simulink model "LongLatDriveline"  (R2024b)
settings: Solver=FixedStepAuto  StartTime=0  StopTime=120  FixedStep=0.002  RelTol=1e-3
InitFcn:
  | load('waypoints.mat');
  | VehicleObj = Simulink.data.dictionary.open('./ModelData/VehicleData.sldd');
  | %dDataSectObj = getSection(myDictionaryObj,'Design Data');
StopFcn:
  | Plot_LateralModelErrorControl;
  | 
  | mdlWks = get_param(gcs, 'ModelWorkspace');
  | par_ToDrvDesigner = evalin(mdlWks, 'ToDrvDesigner');
  | 
  | if par_ToDrvDesigner.Value
  |     ExportdrivingScenario;
  | end
model workspace (MAT data in the model file):
  ToDrvDesigner = Simulink.Parameter
  ToDrvDesigner.Value = 1
  ToDrvDesigner.Complexity = 'real'
  ToDrvDesigner.Dimensions = [1 1]
  ToDrvDesigner.DataType = 'boolean'
values from neighbouring files (symbols this model uses):
  A_F = 2.341157    [VehicleData.sldd]
  C_af = 80000.0    [VehicleData.sldd]
  C_ar = 80000.0    [VehicleData.sldd]
  C_d = 0.24    [VehicleData.sldd]
  f = 0.01    [VehicleData.sldd]
  g = 9.81    [VehicleData.sldd]
  h_aero = 0.65    [VehicleData.sldd]
  h_gc = 0.65    [VehicleData.sldd]
  Iz = 2873.0    [VehicleData.sldd]
  lf = 1.1    [VehicleData.sldd]
  lr = 1.58    [VehicleData.sldd]
  m = 2238.932    [VehicleData.sldd]
  Nf = 2.0    [VehicleData.sldd]
  Nr = 2.0    [VehicleData.sldd]
  r_stat = 0.342    [VehicleData.sldd]
  r_w = 0.352    [VehicleData.sldd]
  rho = 1.225    [VehicleData.sldd]
  theta = 0.0    [VehicleData.sldd]
  transGear = 0.1027    [VehicleData.sldd]
  V_wind = 0.0    [VehicleData.sldd]
undefined symbols (not defined in the file or in its folder): InitialPsi, InitialX, InitialY, phi
libraries: slpidlib x14, spsMosfetLib x6, simulink x4, spsVoltageMeasurementLib x3, SignalEditorBlockLib x2, spsDCVoltageSourceLib x1, spspowerguiLib x1
(part 1 of 5)
settings Model: DataDictionary=VehicleData.sldd  Creator=headl  LastModifiedBy=headl
settings SolverCC: NumberNewtonIterations=3  AlgebraicLoopSolver=TrustRegion
settings DataIOCC: SaveFormat=StructureWithTime  DSMLoggingName=datalog
settings OptimizationCC: BlockReduction=off  BufferReuse=off  ZeroExternalMemoryAtStartup=off  ZeroInternalMemoryAtStartup=off  InitFltsAndDblsToZero=on
settings DebuggingCC: SignalRangeChecking=warning  AlgebraicLoopMsg=none
settings HardwareCC: ProdLongLongMode=on  ProdHWDeviceType=AMD->x86-64 (Windows64)  TargetLongLongMode=on
settings ModelReferenceCC: EnableRefExpFcnMdlSchedulingChecks=on
settings SFSimCC: CustomCodeUndefinedFunction=UseInterfaceOnly  SimTargetLang=C++  SimGPUCompilerFlags=-allow-unsupported-compiler -D_ALLOW_COMPILER_AND_STL_VERSION_MISMATCH
settings RTWCC: TargetLang=C++  GPUComputeCapability=3.5  DLArmComputeVersion=19.05
settings GRTTargetCC: TargetLangStandard=C++11 (ISO)  CodeInterfacePackaging=C++ class

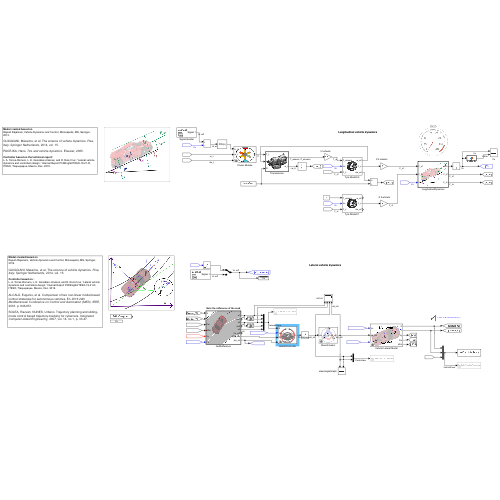
[thumbnail: Simulink's stored preview of the top-level diagram]
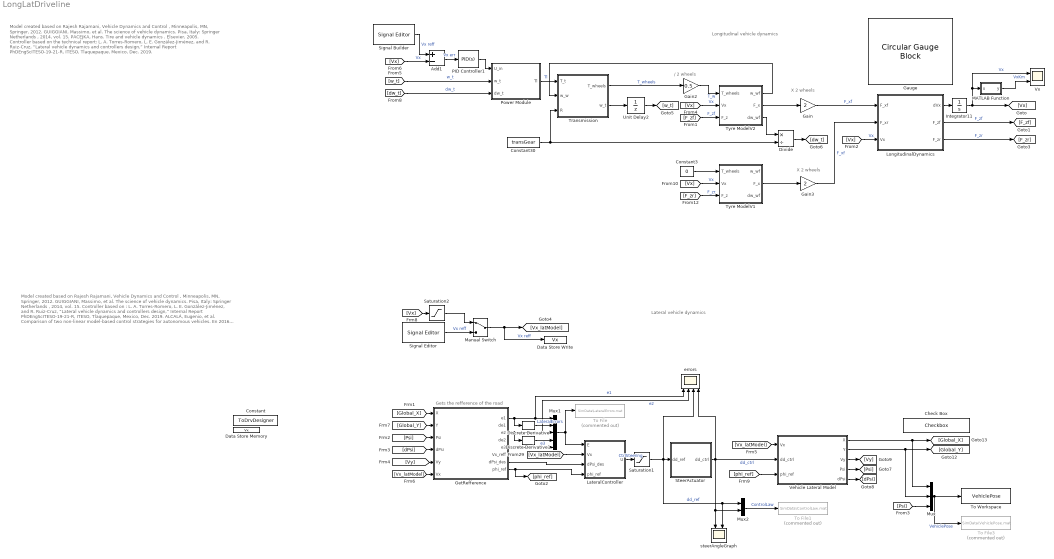
== system LongLatDriveline ==
  note: X 2 wheels
  note: Model created based on
      | Rajesh Rajamani, Vehicle Dynamics and Control , Minneapolis, MN, Springer, 2012.
      |
      | GUIGGIANI, Massimo, et al. The science of vehicle dynamics. Pisa, Italy: Springer Netherlands , 2014, vol. 15.
      |
      | Controller based on :
      | L. A. Torres-Romero, L. E. González-Jiménez, and R. Ruiz-Cruz, “Lateral vehicle dynamics and controllers design,” Internal Report PhDEngScITESO-19-21-R, ITESO, Tlaquepaque, Mexico, Dec. 2019.
      |
      | ALCALÁ, Eugenio, et al. Comparison of two non-linear model-based control strategies for autonomous vehicles. En 2016 24th Mediterranean Conference on Control and Automation (MED) . IEEE, 2016. p. 846-851.
      |
      | SOLEA, Razvan; NUNES, Urbano. Trajectory planning and sliding-mode control based trajectory-tracking for cybercars. Integrated Computer-Aided Engineering , 2007, vol. 14, no 1, p. 33-47.
  note: Gets the refference of the road
  note: Lateral vehicle dynamics
  note: Model created based on
      | Rajesh Rajamani, Vehicle Dynamics and Control , Minneapolis, MN, Springer, 2012.
      |
      | GUIGGIANI, Massimo, et al. The science of vehicle dynamics. Pisa, Italy: Springer Netherlands , 2014, vol. 15.
      |
      | PACEJKA, Hans. Tire and vehicle dynamics . Elsevier, 2005.
      |
      | Controller based on the technical report:
      | L. A. Torres-Romero, L. E. González-Jiménez, and R. Ruiz-Cruz, “Lateral vehicle dynamics and controllers design,” Internal Report PhDEngScITESO-19-21-R, ITESO, Tlaquepaque, Mexico, Dec. 2019.
  note: X 2 wheels
  note: / 2 wheels
  note: Longitudinal vehicle dynamics
  Add1 : Sum  Inputs=+-
  Check Box : Checkbox  LabelPosition=Hide  ShowInitialText=on  Label=To Drv Scenario Designer
  Constant : Constant  Value=ToDrvDesigner
  Constant3 : Constant  Value=0
  Constant30 : Constant  Value=transGear
  Data Store Memory : DataStoreMemory  DataStoreName=Vx  WriteAfterWriteMsg=warning  ShowAdditionalParam=off
  Data Store Write : DataStoreWrite  DataStoreName=Vx  IndexOptions=Index vector (dialog)  Indices=1  OutputSizes=1
  Discrete Derivative : simulink/Discrete/Discrete Derivative  gainval=1.0  ICPrevScaledInput=0.0  OutMin=[]  OutMax=[]  OutDataType=fixdt(1, 16)  OutScaling=2^-10  DoSatur=off
  Discrete Derivative1 : simulink/Discrete/Discrete Derivative  gainval=1.0  ICPrevScaledInput=0.0  OutMin=[]  OutMax=[]  OutDataType=fixdt(1, 16)  OutScaling=2^-10  DoSatur=off
  Divide : Product  Inputs=*/
  Gain : Gain  Gain=2
  Gain2 : Gain  Gain=0.5
  Gain3 : Gain  Gain=2
  Gauge : CircularGaugeBlock  ScaleMax=280  TickInterval=40
  GetRefference : MATLAB Function  TreatAsAtomicUnit=on  SystemSampleTime=0.05
  Integrator11 : Integrator  InitialCondition=0.3
  LateralController : Subsystem  Variant=on  VariantControlMode=label  LabelModeActiveChoice=Ackerman error feedback
      mask Display: image('steeringWheel.png', [0,0,0,0,90,90]);
  LongitudinalDynamics : MATLAB Function  TreatAsAtomicUnit=on
  MATLAB Function : MATLAB Function  TreatAsAtomicUnit=on
  Manual Switch : ManualSwitch
  Mux : Mux  Inputs=3
  Mux1 : Mux  Inputs=5
  Mux2 : Mux  Inputs=2
  PID Controller1 : slpidlib/PID Controller  Controller=PID  Form=Parallel  TimeDomain=Continuous-time  UseExternalTs=off  SampleTime=-1  IntegratorMethod=Forward Euler  FilterMethod=Forward Euler  ControllerParametersSource=internal  P=20  I=0.6  UseKiTs=off  D=100  UseExternalDerivativeSource=off  N=0.0211280216667304  UseFilter=on  TunerSelectOption=Transfer Function Based (PID Tuner App)  InitialConditionSource=internal  InitialConditionForIntegrator=0  InitialConditionForFilter=0  DifferentiatorICPrevScaledInput=0  ExternalReset=none  TrackingMode=off  Kt=1  LimitOutput=off  SatLimitsSource=internal  UpperSaturationLimit=inf  LowerSaturationLimit=-inf  LinearizeAsGain=on  AntiWindupMode=none  Kb=1  LimitIntegrator=off  UpperIntegratorSaturationLimit=inf  LowerIntegratorSaturationLimit=-inf  POutMin=[]  POutMax=[]  IOutMin=[]  IOutMax=[]  DOutMin=[]  DOutMax=[]  NOutMin=[]  NOutMax=[]  SumOutMin=[]  SumOutMax=[]  SaturationOutMin=[]  SaturationOutMax=[]  PParamMin=[]  PParamMax=[]  IParamMin=[]  IParamMax=[]  DParamMin=[]  DParamMax=[]  NParamMin=[]  NParamMax=[]  KbParamMin=[]  KbParamMax=[]  KtParamMin=[]  KtParamMax=[]  KbOutMin=[]  KbOutMax=[]  KtOutMin=[]  KtOutMax=[]  IntegratorOutMin=[]  IntegratorOutMax=[]  FilterOutMin=[]  FilterOutMax=[]  SumI1OutMin=[]  SumI1OutMax=[]  SumI2OutMin=[]  SumI2OutMax=[]  SumI3OutMin=[]  SumI3OutMax=[]  SumI4OutMin=[]  SumI4OutMax=[]  SumDOutMin=[]  SumDOutMax=[]  DifferentiatorOutMin=[]  DifferentiatorOutMax=[]  FilterDiffOutCoefMin=[]  FilterDiffOutCoefMax=[]  ReciprocalOutMin=[]  ReciprocalOutMax=[]  SumDenOutMin=[]  SumDenOutMax=[]  SumNumOutMin=[]  SumNumOutMax=[]  DivideOutMin=[]  DivideOutMax=[]  UdiffTsProdOutMin=[]  UdiffTsProdOutMax=[]  NTsProdOutMin=[]  NTsProdOutMax=[]  UintegralTsProdOutMin=[]  UintegralTsProdOutMax=[]  UngainTsProdOutMin=[]  UngainTsProdOutMax=[]  ClampingZeroOutDataTypeStr=Inherit: Inherit via back propagation  ClampingZeroOutMin=[]  ClampingZeroOutMax=[]  FilterDenConstantOutDataTypeStr=Inherit: Inherit via back propagation  FilterDenConstantOutMin=[]  FilterDenConstantOutMax=[]  PCopyOutDataTypeStr=Inherit: Inherit via back propagation  PCopyOutMin=[]  PCopyOutMax=[]  NCopyOutDataTypeStr=Inherit: Inherit via back propagation  NCopyOutMin=[]  NCopyOutMax=[]  IntegratorContinuousStateAttributes=''  IntegratorStateMustResolveToSignalObject=off  IntegratorRTWStateStorageClass=Auto  FilterContinuousStateAttributes=''  FilterStateMustResolveToSignalObject=off  FilterRTWStateStorageClass=Auto  ParallelPVariant=InternalParameters  IdealPVariant=Disabled  IVariant=InternalParameters  DVariant=InternalParameters  IntegratorVariant=Continuous  SatVariant=Disabled  AWVariant=Passthrough  PCopyVariant=Disabled  TRVariant=Disabled  FdbkBlocksVariant=Forward  IdealPFdbkVariant=Disabled  SatFdbkVariant=Disabled  DerivativeFilterVariant=ContFilter  NVariant=InternalParameters  NCopyVariant=Disabled  FilterICVariant=InternalICsFilter  IntegratorICVariant=InternalICs  ExternalResetVariant=Disabled  TRSumVariant=Passthrough  SumFdbkVariant=Disabled  SumVariant=Sum_PID  TsampFilterVariant=InternalTs  TsampNgainVariant=Passthrough  TsampIntegralVariant=Disabled_SignalSpec  ExternalSaturationOutDataTypeStr=Inherit: Same as second input  DerivativeSourceVariant=ErrorSignal  PreIntVariant=InternalPreInt
  Power Module : Subsystem  Variant=on  VariantControlMode=label  LabelModeActiveChoice=Direct signal
  Saturation1 : Saturate  UpperLimit=pi/4  LowerLimit=-pi/4
  Saturation2 : Saturate  UpperLimit=1000000000  LowerLimit=0.5
  Signal Builder : SignalEditorBlockLib/Signal Editor  FileName=SB_SpeedRef.mat  ActiveScenario=Scenario  ActiveSignal=Signal 1  IsBus=off  OutputBusObjectStr=Bus: BusObject  SampleTime=0  ZeroCross=off  OutputAfterFinalValue=Setting to zero  Unit=inherit  PreserveSignalName=on  ApplySigPropsToAllScenarios=on  ApplySigPropsToAllSignals=off
  Signal Editor : SignalEditorBlockLib/Signal Editor  FileName=LongSpeedProfile.mat  ActiveScenario=Scenario  ActiveSignal=Signal 1  IsBus=off  OutputBusObjectStr=Bus: BusObject  SampleTime=0  ZeroCross=off  OutputAfterFinalValue=Setting to zero  Unit=inherit  PreserveSignalName=on  ApplySigPropsToAllScenarios=on  ApplySigPropsToAllSignals=off
  SteerActuator : Subsystem  Variant=on  VariantControlMode=label  LabelModeActiveChoice=No Actuator
      mask Display: image('motorBLDC.png', [0,0,0,0,95,95]);
  To File : ToFile  Commented=on  Filename=SimData\LateralErrors.mat  SaveFormat=Timeseries
  To File1 : ToFile  Commented=on  Filename=SimData\ControlLaw.mat  SaveFormat=Timeseries
  To File3 : ToFile  Commented=on  Filename=SimData\VehiclePose.mat  SaveFormat=Timeseries
  To Workspace : ToWorkspace  VariableName=VehiclePose  SampleTime=-1
  Transmission : MATLAB Function  TreatAsAtomicUnit=on
  Tyre ModelV1 : Subsystem
      mask Display: image('$imagefile'); % Use "Edit Image" on toolstrip to change.
  Tyre ModelV2 : Subsystem
      mask Display: image('$imagefile'); % Use "Edit Image" on toolstrip to change.
  Unit Delay2 : UnitDelay  SampleTime=-1  HasFrameUpgradeWarning=on
  Vehicle Lateral Model : Subsystem  Variant=on  VariantControlMode=label  LabelModeActiveChoice=Dynamic Model
  Vx : Scope  NumInputPorts=2
  errors : Scope  NumInputPorts=4
  steerAngleGraph : Scope  NumInputPorts=2
  wires:
  Saturation1/1 -> Mux2/1, steerAngleGraph/2, errors/3, SteerActuator/1(dd_ref)  "dd_ref"
  Mux1/1 -> To File/1, LateralController/1(E)  "LateralErrors"
  Mux/1 -> To File3/1, To Workspace/1  "VehiclePose"
  [Global_X] -> GetRefference/1(X)
  [Global_Y] -> GetRefference/2(Y)
  [Psi] -> GetRefference/3(Psi)
  [dPsi] -> GetRefference/4(dPsi)
  [Vy] -> GetRefference/5(Vy)
  [Vx_latModel] -> GetRefference/6(Vx)
  GetRefference/1(e1) -> Discrete Derivative/1, errors/1, Mux1/1  "e1"
  GetRefference/3(e2) -> errors/2, Mux1/3, Discrete Derivative1/1  "e2"
  Divide/1 -> [dw_t]
  Transmission/2(w_t) -> Unit Delay2/1
  Constant30/1 -> Transmission/3(R), Divide/2
  Unit Delay2/1 -> [w_t]
  Tyre ModelV2/3(dw_wf) -> Divide/1
  Tyre ModelV2/2(F_x) -> Gain/1
  Gain/1 -> LongitudinalDynamics/1(F_xf)  "F_xf"
  [Vx] -> Tyre ModelV2/2(Vx)  "Vx"
  [F_zf] -> Tyre ModelV2/3(F_z)  "F_zf"
  Tyre ModelV2/1(w_wf) -> Transmission/2(w_w)
  [dw_t] -> Power Module/3(dw_t)  "dw_t"
  [w_t] -> Power Module/2(w_t)  "w_t"
  LongitudinalDynamics/1(dVx) -> Integrator11/1
  Transmission/1(T_wheels) -> Gain2/1  "T_wheels"
  [Vx] -> LongitudinalDynamics/3(Vx)  "Vx"
  Integrator11/1 -> [Vx], Vx/1, MATLAB Function/1(u)  "Vx"
  Gain2/1 -> Tyre ModelV2/1(T_wheels)  "T_w"
  Constant3/1 -> Tyre ModelV1/1(T_wheels)
  [Vx] -> Tyre ModelV1/2(Vx)  "Vx"
  [F_zr] -> Tyre ModelV1/3(F_z)  "F_zr"
  Tyre ModelV1/2(F_x) -> Gain3/1
  Gain3/1 -> LongitudinalDynamics/2(F_xr)  "F_xf"
  LongitudinalDynamics/2(F_zf) -> [F_zf]  "F_zf"
  LongitudinalDynamics/3(F_zr) -> [F_zr]  "F_zr"
  Power Module/1(Tl) -> Transmission/1(T_t)  "Tl"
  SteerActuator/1(dd_ctrl) -> errors/4, Mux2/2, steerAngleGraph/1, Vehicle Lateral Model/2(dd_ctrl)  "dd_ctrl"
  [Vx] -> Add1/2  "Vx"
  Signal Builder/1 -> Add1/1  "Vx reff"
  [Vx_latModel] -> LateralController/2(Vx)
  LateralController/1(U) -> Saturation1/1  "CtrlSteering"
  [Vx] -> Saturation2/1
  GetRefference/5(e3) -> Mux1/5  "e3"
  Add1/1 -> PID Controller1/1  "Vx err"
  PID Controller1/1 -> Power Module/1(U_in)
  GetRefference/7(dPsi_des) -> LateralController/3(dPsi_des)
  GetRefference/8(phi_ref) -> [phi_ref], LateralController/4(phi_ref)
  Manual Switch/1 -> Data Store Write/1, [Vx_latModel]  "Vx reff"
  [Psi] -> Mux/3
  Mux2/1 -> To File1/1  "ControlLaw"
  Vehicle Lateral Model/1(X) -> Mux/1, [Global_X]
  Vehicle Lateral Model/2(Y) -> Mux/2, [Global_Y]
  [Vx_latModel] -> Vehicle Lateral Model/1(Vx)
  [phi_ref] -> Vehicle Lateral Model/3(phi_ref)
  Vehicle Lateral Model/4(Psi) -> [Psi]
  Vehicle Lateral Model/5(dPsi) -> [dPsi]
  Vehicle Lateral Model/3(Vy) -> [Vy]
  MATLAB Function/1(y) -> Vx/2  "VxKm"
  Discrete Derivative/1 -> Mux1/2
  Discrete Derivative1/1 -> Mux1/4
  Signal Editor/1 -> Manual Switch/2  "Vx reff"
  Saturation2/1 -> Manual Switch/1

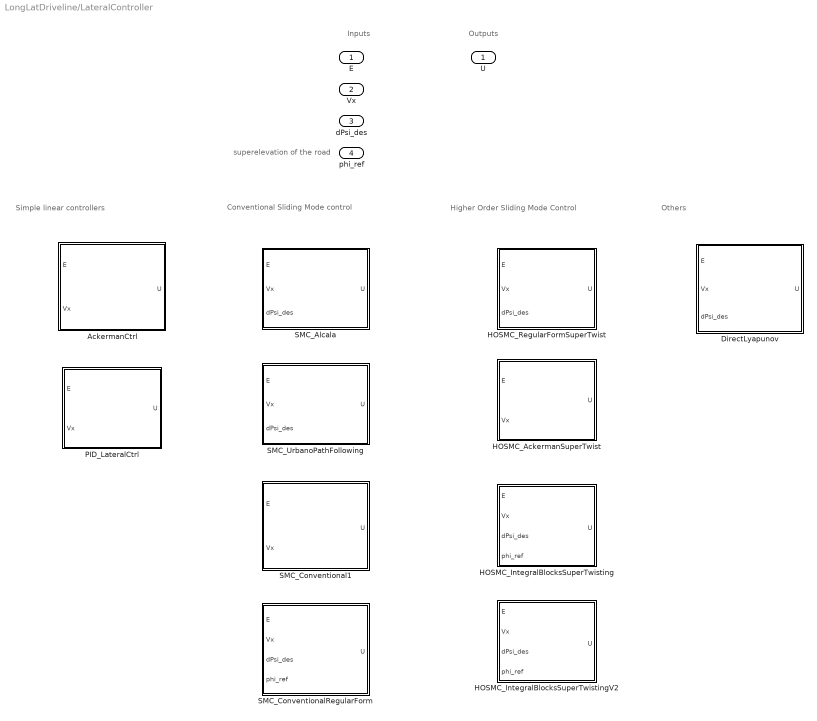
== system LongLatDriveline/LateralController ==
  note: Others
  note: Higher Order Sliding Mode Control
  note: Conventional Sliding Mode control
  note: Simple linear controllers
  note: Outputs
  note: Inputs
  note: superelevation of the road
  E : Inport
  Vx : Inport  Port=2
  dPsi_des : Inport  Port=3
  phi_ref : Inport  Port=4
  AckermanCtrl : MATLAB Function  TreatAsAtomicUnit=on  VariantControl=Ackerman error feedback
  DirectLyapunov : MATLAB Function  TreatAsAtomicUnit=on  VariantControl=Direct Lyapunov Alcala et al.
  HOSMC_AckermanSuperTwist : Subsystem  VariantControl="HOSM  Ackerman + super twisting"
      mask Display: image('$imagefile'); % Use "Edit Image" on toolstrip to change.
  HOSMC_IntegralBlocksSuperTwisting : Subsystem  VariantControl=HOSM Error feedback block +Integral super twisting
      mask Display: image('$imagefile'); % Use "Edit Image" on toolstrip to change.
  HOSMC_IntegralBlocksSuperTwistingV2 : Subsystem  VariantControl=HOSM Block Controller with Integral Super-Twisting Algorithm
      mask Display: image('$imagefile'); % Use "Edit Image" on toolstrip to change.
  HOSMC_RegularFormSuperTwist : Subsystem  VariantControl=HOSM regular form +super twisting
      mask Display: image('$imagefile'); % Use "Edit Image" on toolstrip to change.
  PID_LateralCtrl : Subsystem  VariantControl=PID controller
      mask Display: image('$imagefile'); % Use "Edit Image" on toolstrip to change.
  SMC_Alcala : Subsystem  VariantControl=Sliding mode Alcala et al.
      mask Display: image('$imagefile'); % Use "Edit Image" on toolstrip to change.
  SMC_Conventional1 : MATLAB Function  TreatAsAtomicUnit=on  VariantControl=SMC conventional V1
  SMC_ConventionalRegularForm : MATLAB Function  TreatAsAtomicUnit=on  VariantControl=SMC conventional regular form
  SMC_UrbanoPathFollowing : Subsystem  VariantControl=Sliding mode Urbano path following
      mask Display: image('$imagefile'); % Use "Edit Image" on toolstrip to change.
  U : Outport

== system LongLatDriveline/Power Module ==
  U_in : Inport
  w_t : Inport  Port=2
  dw_t : Inport  Port=3
  BLDC Motor : Subsystem  Variant=on  VariantControlMode=label  VariantControl=BLDC Motor  LabelModeActiveChoice=BLDC dq Model
      mask Display: image('BLDC.jpg');
  DC Motor : Subsystem  VariantControl=DC_Motor
      mask Display: image('BLDC.jpg');
  SIEngineModel : Subsystem  VariantControl=SI Engine
      mask Display: image('BLDC.jpg');
  SignalBuilder : Subsystem  VariantControl=Direct signal
      mask Display: image('BLDC.jpg');
  Tl : Outport

== system LongLatDriveline/SteerActuator ==
  dd_ref : Inport
  BLDCWRack : Subsystem  VariantControl=BLDCWRack
      mask Display: image('BLDC_1.jpg');
  BLDC_AngleCtrl : Subsystem  VariantControl=BLDC electric motor  mask{lambda=0.0333, R=0.08, L=0.0001, M=0, J=0.00018, b=0.00034, P=8}
      mask prompts: lambda "BEMF factor ........................"; R "Phase resistance (R)..............."; L "Phase inductance (L)...."; M "Mutual inductance (M).........."; J "Rotor inertia (J)......................."; b "Viscous friction (b)................."; P "Poles qty (P).............................."
      mask Display: image('$imagefile'); % Use "Edit Image" on toolstrip to change.
  NoActuator : Subsystem  VariantControl=No Actuator
  genericTransferFunction : Subsystem  VariantControl=Generic transfer function
      mask Display: image('$imagefile'); % Use "Edit Image" on toolstrip to change.
  dd_ctrl : Outport

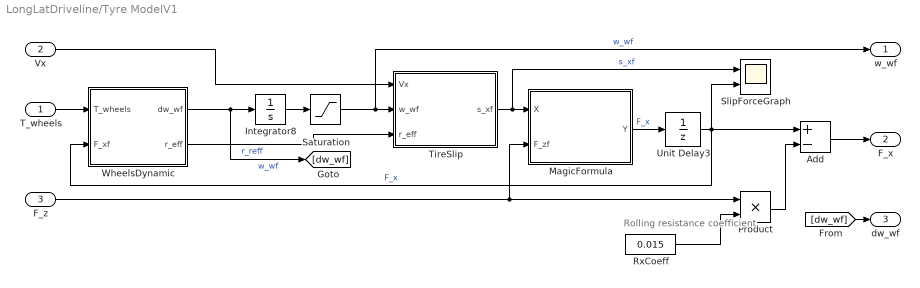
== system LongLatDriveline/Tyre ModelV1 ==
  note: Rolling resistance
      | coefficient
  T_wheels : Inport
  Vx : Inport  Port=2
  F_z : Inport  Port=3
  Add : Sum  Inputs=+-
  Integrator8 : Integrator
  MagicFormula : MATLAB Function  TreatAsAtomicUnit=on
  Product : Product
  RxCoeff : Constant  Value=0.015
  Saturation : Saturate  UpperLimit=100000  LowerLimit=0
  SlipForceGraph : Scope  NumInputPorts=2
  TireSlip : MATLAB Function  TreatAsAtomicUnit=on
  Unit Delay3 : UnitDelay  SampleTime=-1  HasFrameUpgradeWarning=on
  WheelsDynamic : MATLAB Function  TreatAsAtomicUnit=on
  w_wf : Outport
  F_x : Outport  Port=2
  dw_wf : Outport  Port=3
  wires:
  T_wheels/1 -> WheelsDynamic/1(T_wheels)
  Saturation/1 -> w_wf/1, TireSlip/2(w_wf)  "w_wf"
  WheelsDynamic/2(r_eff) -> TireSlip/3(r_eff)  "r_reff"
  MagicFormula/1(Y) -> Unit Delay3/1  "F_x"
  TireSlip/1(s_xf) -> SlipForceGraph/1, MagicFormula/1(X)  "s_xf"
  Integrator8/1 -> Saturation/1
  Vx/1 -> TireSlip/1(Vx)
  [dw_wf] -> dw_wf/1
  WheelsDynamic/1(dw_wf) -> [dw_wf], Integrator8/1  "w_wf"
  Add/1 -> F_x/1
  Product/1 -> Add/2
  F_z/1 -> Product/1, MagicFormula/2(F_zf)
  Unit Delay3/1 -> Add/1, SlipForceGraph/2, WheelsDynamic/2(F_xf)  "F_x"
  RxCoeff/1 -> Product/2

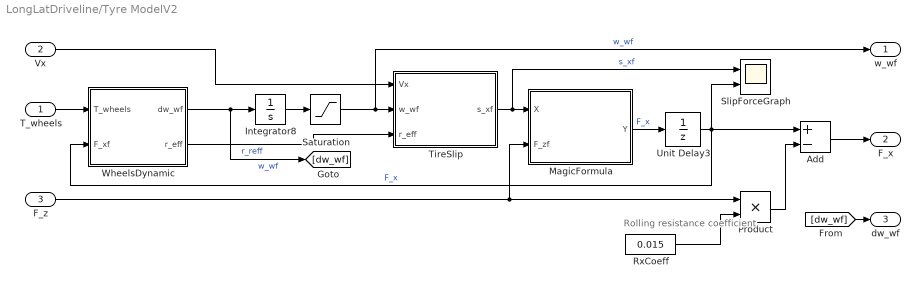
== system LongLatDriveline/Tyre ModelV2 ==
  note: Rolling resistance
      | coefficient
  T_wheels : Inport
  Vx : Inport  Port=2
  F_z : Inport  Port=3
  Add : Sum  Inputs=+-
  Integrator8 : Integrator
  MagicFormula : MATLAB Function  TreatAsAtomicUnit=on
  Product : Product
  RxCoeff : Constant  Value=0.015
  Saturation : Saturate  UpperLimit=100000  LowerLimit=0
  SlipForceGraph : Scope  NumInputPorts=2
  TireSlip : MATLAB Function  TreatAsAtomicUnit=on
  Unit Delay3 : UnitDelay  SampleTime=-1  HasFrameUpgradeWarning=on
  WheelsDynamic : MATLAB Function  TreatAsAtomicUnit=on
  w_wf : Outport
  F_x : Outport  Port=2
  dw_wf : Outport  Port=3
  wires:
  T_wheels/1 -> WheelsDynamic/1(T_wheels)
  Saturation/1 -> w_wf/1, TireSlip/2(w_wf)  "w_wf"
  WheelsDynamic/2(r_eff) -> TireSlip/3(r_eff)  "r_reff"
  MagicFormula/1(Y) -> Unit Delay3/1  "F_x"
  TireSlip/1(s_xf) -> SlipForceGraph/1, MagicFormula/1(X)  "s_xf"
  Integrator8/1 -> Saturation/1
  Vx/1 -> TireSlip/1(Vx)
  [dw_wf] -> dw_wf/1
  WheelsDynamic/1(dw_wf) -> [dw_wf], Integrator8/1  "w_wf"
  Add/1 -> F_x/1
  Product/1 -> Add/2
  F_z/1 -> Product/1, MagicFormula/2(F_zf)
  Unit Delay3/1 -> Add/1, SlipForceGraph/2, WheelsDynamic/2(F_xf)  "F_x"
  RxCoeff/1 -> Product/2

== system LongLatDriveline/Vehicle Lateral Model ==
  Vx : Inport
  dd_ctrl : Inport  Port=2
  phi_ref : Inport  Port=3
  DynamicModel : Subsystem  VariantControl=Dynamic Model
      mask Display: image('CarBicycleModelDyna.png');
  KinematicModel : Subsystem  VariantControl=Kinematic Model
      mask Display: image('CarBicycleModelKine.png');
  X : Outport
  Y : Outport  Port=2
  Vy : Outport  Port=3
  Psi : Outport  Port=4
  dPsi : Outport  Port=5

== system LongLatDriveline/LateralController/HOSMC_AckermanSuperTwist ==
  E : Inport
  Vx : Inport  Port=2
  HOSMC_AckermanSuperTwis1 : MATLAB Function  TreatAsAtomicUnit=on  VariantControl=SMC conventional
  Integrator1 : Integrator
  U : Outport
  wires:
  HOSMC_AckermanSuperTwis1/1(U) -> U/1
  E/1 -> HOSMC_AckermanSuperTwis1/1(E)
  Vx/1 -> HOSMC_AckermanSuperTwis1/2(Vx)
  HOSMC_AckermanSuperTwis1/2(dMu1) -> Integrator1/1
  Integrator1/1 -> HOSMC_AckermanSuperTwis1/3(Mu1)

== system LongLatDriveline/LateralController/HOSMC_IntegralBlocksSuperTwisting ==
  E : Inport
  Vx : Inport  Port=2
  dPsi_des : Inport  Port=3
  phi_ref : Inport  Port=4
  HOSMC_SuperTwisting : MATLAB Function  TreatAsAtomicUnit=on  VariantControl=SMC conventional
  Integrator1 : Integrator
  Integrator4 : Integrator  LimitOutput=on  UpperSaturationLimit=pi  LowerSaturationLimit=-pi
  MATLAB Function2 : MATLAB Function  TreatAsAtomicUnit=on
  Scope : Scope  NumInputPorts=4
  U : Outport
  wires:
  HOSMC_SuperTwisting/1(U) -> Scope/1, U/1  "U"
  E/1 -> HOSMC_SuperTwisting/1(E)
  Vx/1 -> HOSMC_SuperTwisting/2(Vx)
  HOSMC_SuperTwisting/4(dv) -> Scope/4, Integrator1/1  "dv"
  Integrator1/1 -> HOSMC_SuperTwisting/5(v)  "v"
  dPsi_des/1 -> HOSMC_SuperTwisting/3(dPsi_des)
  phi_ref/1 -> HOSMC_SuperTwisting/4(phi_ref)
  HOSMC_SuperTwisting/3(d_u) -> Scope/3  "d_u"
  HOSMC_SuperTwisting/2(d_k) -> Scope/2  "d_k"
  HOSMC_SuperTwisting/5(de_bn) -> Integrator4/1
  Integrator4/1 -> MATLAB Function2/1(u)  "e_bn"
  MATLAB Function2/1(y) -> HOSMC_SuperTwisting/6(e_bn)  "v"

== system LongLatDriveline/LateralController/HOSMC_IntegralBlocksSuperTwistingV2 ==
  E : Inport
  Vx : Inport  Port=2
  dPsi_des : Inport  Port=3
  phi_ref : Inport  Port=4
  Demux : Demux  Outputs=2
  Demux1 : Demux  Outputs=2
  HOSMC_SuperTwistingV2 : MATLAB Function  TreatAsAtomicUnit=on  VariantControl=SMC conventional
  Integrator1 : Integrator  InitialCondition=[0;0]  UpperSaturationLimit=pi  LowerSaturationLimit=-pi
  Integrator2 : Integrator  InitialCondition=[0;0]  UpperSaturationLimit=pi  LowerSaturationLimit=-pi
  Integrator4 : Integrator  InitialCondition=[0;0]  UpperSaturationLimit=pi  LowerSaturationLimit=-pi
  Scope1 : Scope  NumInputPorts=3
  Scope2 : Scope  NumInputPorts=3
  U : Outport
  wires:
  HOSMC_SuperTwistingV2/1(U) -> U/1  "U"
  E/1 -> HOSMC_SuperTwistingV2/1(E)
  Vx/1 -> HOSMC_SuperTwistingV2/2(Vx)
  dPsi_des/1 -> HOSMC_SuperTwistingV2/3(dPsi_des)
  phi_ref/1 -> HOSMC_SuperTwistingV2/4(phi_ref)
  HOSMC_SuperTwistingV2/2(dz) -> Integrator4/1  "dz"
  Integrator4/1 -> HOSMC_SuperTwistingV2/5(z)  "z"
  HOSMC_SuperTwistingV2/4(dv1) -> Demux1/1, Integrator1/1
  Integrator1/1 -> HOSMC_SuperTwistingV2/7(v1)  "v1"
  HOSMC_SuperTwistingV2/3(dv0) -> Integrator2/1, Demux/1
  Integrator2/1 -> HOSMC_SuperTwistingV2/6(v0)  "v2"
  Demux/2 -> Scope1/2  "dv0_psie"
  HOSMC_SuperTwistingV2/5(d_0) -> Scope1/3  "d_0"
  Demux/1 -> Scope1/1  "dv0_ye"
  HOSMC_SuperTwistingV2/6(d_1) -> Scope2/3  "d_1"
  Demux1/1 -> Scope2/1  "dv1_ye"
  Demux1/2 -> Scope2/2  "dv1_psie"

== system LongLatDriveline/LateralController/HOSMC_RegularFormSuperTwist ==
  E : Inport
  Vx : Inport  Port=2
  dPsi_des : Inport  Port=3
  HOSMC_RegularFormSuperTwist : MATLAB Function  TreatAsAtomicUnit=on  VariantControl=SMC conventional
  Integrator1 : Integrator
  Scope : Scope  NumInputPorts=3
  U : Outport
  wires:
  HOSMC_RegularFormSuperTwist/1(U) -> Scope/1, U/1
  E/1 -> HOSMC_RegularFormSuperTwist/1(E)
  Vx/1 -> HOSMC_RegularFormSuperTwist/2(Vx)
  HOSMC_RegularFormSuperTwist/2(dMu1) -> Integrator1/1, Scope/2
  Integrator1/1 -> Scope/3, HOSMC_RegularFormSuperTwist/4(Mu1)
  dPsi_des/1 -> HOSMC_RegularFormSuperTwist/3(dPsi_des)

== system LongLatDriveline/LateralController/PID_LateralCtrl ==
  note: Sum of the normalized errors. assuming max orientation error as pi, and 12ft as max error respect the center of the lane.
  note: assumming pi as maximum error orientation
  note: 12 ft aprx width of a lane.
  E : Inport
  Vx : Inport  Port=2
  Constant : Constant  Value=pi
  Constant1 : Constant  Value=3.6576
  Demux : Demux  Outputs=5
  Divide : Product  Inputs=*/
  Divide1 : Product  Inputs=*/
  PID Controller : slpidlib/PID Controller  Controller=PID  Form=Parallel  TimeDomain=Continuous-time  UseExternalTs=off  SampleTime=-1  IntegratorMethod=Forward Euler  FilterMethod=Forward Euler  ControllerParametersSource=internal  P=-1.07026319725058  I=-0.0114731538990864  UseKiTs=off  D=-13.315697744938  UseExternalDerivativeSource=off  N=0.137087779250562  UseFilter=on  TunerSelectOption=Transfer Function Based (PID Tuner App)  InitialConditionSource=internal  InitialConditionForIntegrator=0  InitialConditionForFilter=0  DifferentiatorICPrevScaledInput=0  ExternalReset=none  TrackingMode=off  Kt=1  LimitOutput=off  SatLimitsSource=internal  UpperSaturationLimit=inf  LowerSaturationLimit=-inf  LinearizeAsGain=on  AntiWindupMode=none  Kb=1  LimitIntegrator=off  UpperIntegratorSaturationLimit=inf  LowerIntegratorSaturationLimit=-inf  POutMin=[]  POutMax=[]  IOutMin=[]  IOutMax=[]  DOutMin=[]  DOutMax=[]  NOutMin=[]  NOutMax=[]  SumOutMin=[]  SumOutMax=[]  SaturationOutMin=[]  SaturationOutMax=[]  PParamMin=[]  PParamMax=[]  IParamMin=[]  IParamMax=[]  DParamMin=[]  DParamMax=[]  NParamMin=[]  NParamMax=[]  KbParamMin=[]  KbParamMax=[]  KtParamMin=[]  KtParamMax=[]  KbOutMin=[]  KbOutMax=[]  KtOutMin=[]  KtOutMax=[]  IntegratorOutMin=[]  IntegratorOutMax=[]  FilterOutMin=[]  FilterOutMax=[]  SumI1OutMin=[]  SumI1OutMax=[]  SumI2OutMin=[]  SumI2OutMax=[]  SumI3OutMin=[]  SumI3OutMax=[]  SumI4OutMin=[]  SumI4OutMax=[]  SumDOutMin=[]  SumDOutMax=[]  DifferentiatorOutMin=[]  DifferentiatorOutMax=[]  FilterDiffOutCoefMin=[]  FilterDiffOutCoefMax=[]  ReciprocalOutMin=[]  ReciprocalOutMax=[]  SumDenOutMin=[]  SumDenOutMax=[]  SumNumOutMin=[]  SumNumOutMax=[]  DivideOutMin=[]  DivideOutMax=[]  UdiffTsProdOutMin=[]  UdiffTsProdOutMax=[]  NTsProdOutMin=[]  NTsProdOutMax=[]  UintegralTsProdOutMin=[]  UintegralTsProdOutMax=[]  UngainTsProdOutMin=[]  UngainTsProdOutMax=[]  ClampingZeroOutDataTypeStr=Inherit: Inherit via back propagation  ClampingZeroOutMin=[]  ClampingZeroOutMax=[]  FilterDenConstantOutDataTypeStr=Inherit: Inherit via back propagation  FilterDenConstantOutMin=[]  FilterDenConstantOutMax=[]  PCopyOutDataTypeStr=Inherit: Inherit via back propagation  PCopyOutMin=[]  PCopyOutMax=[]  NCopyOutDataTypeStr=Inherit: Inherit via back propagation  NCopyOutMin=[]  NCopyOutMax=[]  IntegratorContinuousStateAttributes=''  IntegratorStateMustResolveToSignalObject=off  IntegratorRTWStateStorageClass=Auto  FilterContinuousStateAttributes=''  FilterStateMustResolveToSignalObject=off  FilterRTWStateStorageClass=Auto  ParallelPVariant=InternalParameters  IdealPVariant=Disabled  IVariant=InternalParameters  DVariant=InternalParameters  IntegratorVariant=Continuous  SatVariant=Disabled  AWVariant=Passthrough  PCopyVariant=Disabled  TRVariant=Disabled  FdbkBlocksVariant=Forward  IdealPFdbkVariant=Disabled  SatFdbkVariant=Disabled  DerivativeFilterVariant=ContFilter  NVariant=InternalParameters  NCopyVariant=Disabled  FilterICVariant=InternalICsFilter  IntegratorICVariant=InternalICs  ExternalResetVariant=Disabled  TRSumVariant=Passthrough  SumFdbkVariant=Disabled  SumVariant=Sum_PID  TsampFilterVariant=InternalTs  TsampNgainVariant=Passthrough  TsampIntegralVariant=Disabled_SignalSpec  ExternalSaturationOutDataTypeStr=Inherit: Same as second input  DerivativeSourceVariant=ErrorSignal  PreIntVariant=InternalPreInt
  Subtract : Sum
  Terminator{,1..3} (4 alike) : Terminator
  U : Outport
  wires:
  E/1 -> Demux/1
  Demux/2 -> Terminator/1  "de1"
  Demux/4 -> Terminator2/1  "de2"
  Vx/1 -> Terminator3/1
  Demux/3 -> Divide/1  "e2"
  Divide/1 -> Subtract/2
  Constant/1 -> Divide/2
  Demux/1 -> Divide1/1  "e1"
  Constant1/1 -> Divide1/2
  Divide1/1 -> Subtract/1
  Demux/5 -> Terminator1/1
  PID Controller/1 -> U/1
  Subtract/1 -> PID Controller/1

== system LongLatDriveline/LateralController/SMC_Alcala ==
  note: the derivative of the x error and the angular acceleration in the orientation were obtained using a levant differentiator.
  E : Inport
  Vx : Inport  Port=2
  dPsi_des : Inport  Port=3
  AlcalaSMC : MATLAB Function  TreatAsAtomicUnit=on  VariantControl=Sliding mode Ctrl 1
  Demux : Demux  Outputs=5
  LevantDiff : Subsystem  mask{lambda1=60, alpha1=2000}
      mask prompts: lambda1 "Lambda :"; alpha1 "Alpha    :"
      mask help: Levant differenciator
      mask Help: This is based on Levant A. (1998). Robust exact differentiation via sliding mode technique. Automatica, 34(3), 379-384
  LevantDiff1 : Subsystem  mask{lambda1=60, alpha1=2000}
      mask prompts: lambda1 "Lambda :"; alpha1 "Alpha    :"
      mask help: Levant differenciator
      mask Help: This is based on Levant A. (1998). Robust exact differentiation via sliding mode technique. Automatica, 34(3), 379-384
  Terminator{,1..3} (4 alike) : Terminator
  U : Outport
  wires:
  E/1 -> Demux/1, AlcalaSMC/1(E)
  Vx/1 -> AlcalaSMC/2(Vx)
  dPsi_des/1 -> LevantDiff1/1(X), AlcalaSMC/3(dPsi_des)
  AlcalaSMC/1(U) -> U/1
  Demux/1 -> Terminator/1
  Demux/2 -> Terminator1/1
  Demux/3 -> Terminator2/1
  Demux/4 -> Terminator3/1
  LevantDiff/1(dX) -> AlcalaSMC/4(dx_e)
  Demux/5 -> LevantDiff/1(X)
  LevantDiff1/1(dX) -> AlcalaSMC/5(ddPsi_des)

== system LongLatDriveline/LateralController/SMC_UrbanoPathFollowing ==
  E : Inport
  Vx : Inport  Port=2
  dPsi_des : Inport  Port=3
  Integrator : Integrator
  SMC_UrbanoPathFollowing : MATLAB Function  TreatAsAtomicUnit=on  VariantControl=Sliding mode Urbano Path Following
  U : Outport
  wires:
  SMC_UrbanoPathFollowing/1(U) -> U/1
  E/1 -> SMC_UrbanoPathFollowing/1(E)
  Vx/1 -> SMC_UrbanoPathFollowing/2(Vx)
  dPsi_des/1 -> SMC_UrbanoPathFollowing/3(dPsi_des)
  SMC_UrbanoPathFollowing/2(dd_d) -> Integrator/1
  Integrator/1 -> SMC_UrbanoPathFollowing/4(d_d)

== system LongLatDriveline/Power Module/BLDC Motor ==
  U_in : Inport
  w_t : Inport  Port=2
  dw_t : Inport  Port=3
  BLDC  SVPWM : Subsystem  VariantControl=BLDC SVPWM
      mask Display: image('BLDC.jpg');
  BLDC abcModel : Subsystem  VariantControl=BLDC abc Model
      mask Display: image('BLDC.jpg');
  BLDC dqControl : Subsystem  VariantControl=BLDC dq Model
      mask Display: image('BLDC.jpg');
  Tl : Outport

== system LongLatDriveline/Power Module/DC Motor ==
  U_in : Inport
  w_t : Inport  Port=2
  dw_t : Inport  Port=3
  DC Motor : MATLAB Function  TreatAsAtomicUnit=on
  Integrator4 : Integrator
  Mux : Mux  Inputs=3
  Tl : Outport
  wires:
  dw_t/1 -> Mux/3
  DC Motor/1(dX) -> Integrator4/1
  Integrator4/1 -> DC Motor/1(X)
  Mux/1 -> DC Motor/2(u)
  w_t/1 -> Mux/2
  U_in/1 -> Mux/1
  DC Motor/2(T) -> Tl/1

== system LongLatDriveline/Power Module/SIEngineModel ==
  note: kelvin temp
  note: .8 bar (hendricks)
  U_in : Inport
  w_t : Inport  Port=2
  dw_t : Inport  Port=3
  Constant1 : Constant  Value=373
  Constant2 : Constant  Value=80000
  SI_Engine : Subsystem
  Tl : Outport
  wires:
  Constant2/1 -> SI_Engine/1(p_man)
  Constant1/1 -> SI_Engine/2(T_man)
  U_in/1 -> SI_Engine/3(alpha)
  w_t/1 -> SI_Engine/4(w_e)
  dw_t/1 -> SI_Engine/5(dw_e)
  SI_Engine/1(T_p) -> Tl/1

== system LongLatDriveline/Power Module/SignalBuilder ==
  U_in : Inport
  w_t : Inport  Port=2
  dw_t : Inport  Port=3
  Tl : Outport
  wires:
  U_in/1 -> Tl/1

== system LongLatDriveline/SteerActuator/BLDCWRack ==
  dd_ref : Inport
  BLDC_AngleCtrl2 : Subsystem  VariantControl=BLDC electric motor  mask{lambda=0.0333, R=0.08, L=0.0001, M=0, J=0.00018, b=0.00034, P=8}
      mask prompts: lambda "BEMF factor ........................"; R "Phase resistance (R)..............."; L "Phase inductance (L)...."; M "Mutual inductance (M).........."; J "Rotor inertia (J)......................."; b "Viscous friction (b)................."; P "Poles qty (P).............................."
      mask Display: image('$imagefile'); % Use "Edit Image" on toolstrip to change.
  Constant2 : Constant  Value=4
  Data Store Read : DataStoreRead  DataStoreName=Vx  IndexOptions=Index vector (dialog)  Indices=1  OutputSizes=1
  Product3 : Product
  RackSubsystem : Subsystem
  Tl : Scope  Commented=on
  Unit Delay1 : UnitDelay  SampleTime=-1  HasFrameUpgradeWarning=on
  dd_ctrl : Outport
  wires:
  dd_ref/1 -> Product3/1  "dd_ref"
  RackSubsystem/2(Tl) -> Tl/1, Unit Delay1/1  "Tl"
  BLDC_AngleCtrl2/1(theta_m) -> RackSubsystem/1(theta_m)  "theta_m"
  BLDC_AngleCtrl2/2(dWm) -> RackSubsystem/2(dWm)  "Theta_e"
  BLDC_AngleCtrl2/3(Wm) -> RackSubsystem/3(Wm)  "Wm"
  Unit Delay1/1 -> BLDC_AngleCtrl2/2(Tl)
  Constant2/1 -> Product3/2, RackSubsystem/4(gearboxRate)
  RackSubsystem/1(dd) -> dd_ctrl/1
  Product3/1 -> BLDC_AngleCtrl2/1(dd_ref)
  Data Store Read/1 -> RackSubsystem/5(Vx)

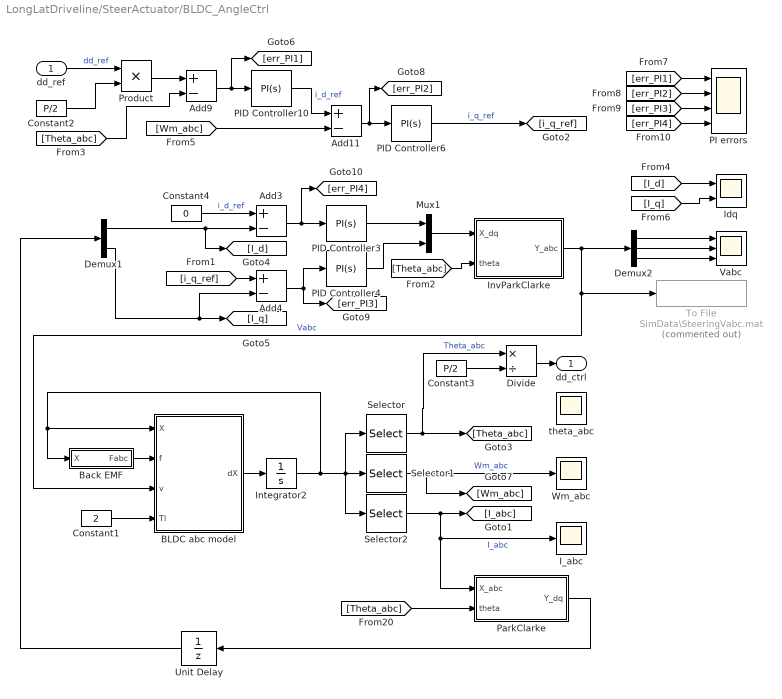
== system LongLatDriveline/SteerActuator/BLDC_AngleCtrl ==
  dd_ref : Inport
  Add{3..4,9,11} (4 alike) : Sum  Inputs=+-
  BLDC abc model : MATLAB Function  TreatAsAtomicUnit=on
  Back EMF : MATLAB Function  TreatAsAtomicUnit=on
  Constant1 : Constant  Value=2
  Constant2 : Constant  Value=P/2
  Constant3 : Constant  Value=P/2
  Constant4 : Constant  Value=0
  Demux1 : Demux  Outputs=2
  Demux2 : Demux  Outputs=3
  Divide : Product  Inputs=*/
  I_abc : Scope
  Idq : Scope  NumInputPorts=2
  Integrator2 : Integrator  InitialCondition=[0;0;0;0.1;0]
  InvParkClarke : MATLAB Function  TreatAsAtomicUnit=on
  Mux1 : Mux  Inputs=2
  PI errors : Scope  NumInputPorts=4
  PID Controller10 : slpidlib/PID Controller  Controller=PI  Form=Parallel  TimeDomain=Continuous-time  UseExternalTs=off  SampleTime=-1  IntegratorMethod=Forward Euler  FilterMethod=Forward Euler  ControllerParametersSource=internal  P=50  I=2  UseKiTs=off  D=0  UseExternalDerivativeSource=off  N=100  UseFilter=on  TunerSelectOption=Transfer Function Based (PID Tuner App)  InitialConditionSource=internal  InitialConditionForIntegrator=0  InitialConditionForFilter=0  DifferentiatorICPrevScaledInput=0  ExternalReset=none  TrackingMode=off  Kt=1  LimitOutput=off  SatLimitsSource=internal  UpperSaturationLimit=500  LowerSaturationLimit=-500  LinearizeAsGain=on  AntiWindupMode=back-calculation  Kb=1  LimitIntegrator=off  UpperIntegratorSaturationLimit=inf  LowerIntegratorSaturationLimit=-inf  POutMin=[]  POutMax=[]  IOutMin=[]  IOutMax=[]  DOutMin=[]  DOutMax=[]  NOutMin=[]  NOutMax=[]  SumOutMin=[]  SumOutMax=[]  SaturationOutMin=[]  SaturationOutMax=[]  PParamMin=[]  PParamMax=[]  IParamMin=[]  IParamMax=[]  DParamMin=[]  DParamMax=[]  NParamMin=[]  NParamMax=[]  KbParamMin=[]  KbParamMax=[]  KtParamMin=[]  KtParamMax=[]  KbOutMin=[]  KbOutMax=[]  KtOutMin=[]  KtOutMax=[]  IntegratorOutMin=[]  IntegratorOutMax=[]  FilterOutMin=[]  FilterOutMax=[]  SumI1OutMin=[]  SumI1OutMax=[]  SumI2OutMin=[]  SumI2OutMax=[]  SumI3OutMin=[]  SumI3OutMax=[]  SumI4OutMin=[]  SumI4OutMax=[]  SumDOutMin=[]  SumDOutMax=[]  DifferentiatorOutMin=[]  DifferentiatorOutMax=[]  FilterDiffOutCoefMin=[]  FilterDiffOutCoefMax=[]  ReciprocalOutMin=[]  ReciprocalOutMax=[]  SumDenOutMin=[]  SumDenOutMax=[]  SumNumOutMin=[]  SumNumOutMax=[]  DivideOutMin=[]  DivideOutMax=[]  UdiffTsProdOutMin=[]  UdiffTsProdOutMax=[]  NTsProdOutMin=[]  NTsProdOutMax=[]  UintegralTsProdOutMin=[]  UintegralTsProdOutMax=[]  UngainTsProdOutMin=[]  UngainTsProdOutMax=[]  ClampingZeroOutDataTypeStr=Inherit: Inherit via back propagation  ClampingZeroOutMin=[]  ClampingZeroOutMax=[]  FilterDenConstantOutDataTypeStr=Inherit: Inherit via back propagation  FilterDenConstantOutMin=[]  FilterDenConstantOutMax=[]  PCopyOutDataTypeStr=Inherit: Inherit via back propagation  PCopyOutMin=[]  PCopyOutMax=[]  NCopyOutDataTypeStr=Inherit: Inherit via back propagation  NCopyOutMin=[]  NCopyOutMax=[]  IntegratorContinuousStateAttributes=''  IntegratorStateMustResolveToSignalObject=off  IntegratorRTWStateStorageClass=Auto  FilterContinuousStateAttributes=''  FilterStateMustResolveToSignalObject=off  FilterRTWStateStorageClass=Auto  ParallelPVariant=InternalParameters  IdealPVariant=Disabled  IVariant=InternalParameters  DVariant=Disabled  IntegratorVariant=Continuous  SatVariant=Disabled  AWVariant=Passthrough  PCopyVariant=Disabled  TRVariant=Disabled  FdbkBlocksVariant=Forward  IdealPFdbkVariant=Disabled  SatFdbkVariant=Disabled  DerivativeFilterVariant=Disabled  NVariant=Disabled  NCopyVariant=Disabled_SignalSpec  FilterICVariant=Disabled  IntegratorICVariant=InternalICs  ExternalResetVariant=Disabled  TRSumVariant=Passthrough  SumFdbkVariant=Disabled  SumVariant=Sum_PI  TsampFilterVariant=InternalTs  TsampNgainVariant=Passthrough  TsampIntegralVariant=Disabled_SignalSpec  ExternalSaturationOutDataTypeStr=Inherit: Same as second input  DerivativeSourceVariant=Disabled  PreIntVariant=InternalPreInt
  PID Controller3 : slpidlib/PID Controller  Controller=PI  Form=Parallel  TimeDomain=Continuous-time  UseExternalTs=off  SampleTime=-1  IntegratorMethod=Forward Euler  FilterMethod=Forward Euler  ControllerParametersSource=internal  P=30  I=0  UseKiTs=off  D=0  UseExternalDerivativeSource=off  N=100  UseFilter=on  TunerSelectOption=Transfer Function Based (PID Tuner App)  InitialConditionSource=internal  InitialConditionForIntegrator=0  InitialConditionForFilter=0  DifferentiatorICPrevScaledInput=0  ExternalReset=none  TrackingMode=off  Kt=1  LimitOutput=off  SatLimitsSource=internal  UpperSaturationLimit=120  LowerSaturationLimit=-120  LinearizeAsGain=on  AntiWindupMode=back-calculation  Kb=1  LimitIntegrator=off  UpperIntegratorSaturationLimit=inf  LowerIntegratorSaturationLimit=-inf  POutMin=[]  POutMax=[]  IOutMin=[]  IOutMax=[]  DOutMin=[]  DOutMax=[]  NOutMin=[]  NOutMax=[]  SumOutMin=[]  SumOutMax=[]  SaturationOutMin=[]  SaturationOutMax=[]  PParamMin=[]  PParamMax=[]  IParamMin=[]  IParamMax=[]  DParamMin=[]  DParamMax=[]  NParamMin=[]  NParamMax=[]  KbParamMin=[]  KbParamMax=[]  KtParamMin=[]  KtParamMax=[]  KbOutMin=[]  KbOutMax=[]  KtOutMin=[]  KtOutMax=[]  IntegratorOutMin=[]  IntegratorOutMax=[]  FilterOutMin=[]  FilterOutMax=[]  SumI1OutMin=[]  SumI1OutMax=[]  SumI2OutMin=[]  SumI2OutMax=[]  SumI3OutMin=[]  SumI3OutMax=[]  SumI4OutMin=[]  SumI4OutMax=[]  SumDOutMin=[]  SumDOutMax=[]  DifferentiatorOutMin=[]  DifferentiatorOutMax=[]  FilterDiffOutCoefMin=[]  FilterDiffOutCoefMax=[]  ReciprocalOutMin=[]  ReciprocalOutMax=[]  SumDenOutMin=[]  SumDenOutMax=[]  SumNumOutMin=[]  SumNumOutMax=[]  DivideOutMin=[]  DivideOutMax=[]  UdiffTsProdOutMin=[]  UdiffTsProdOutMax=[]  NTsProdOutMin=[]  NTsProdOutMax=[]  UintegralTsProdOutMin=[]  UintegralTsProdOutMax=[]  UngainTsProdOutMin=[]  UngainTsProdOutMax=[]  ClampingZeroOutDataTypeStr=Inherit: Inherit via back propagation  ClampingZeroOutMin=[]  ClampingZeroOutMax=[]  FilterDenConstantOutDataTypeStr=Inherit: Inherit via back propagation  FilterDenConstantOutMin=[]  FilterDenConstantOutMax=[]  PCopyOutDataTypeStr=Inherit: Inherit via back propagation  PCopyOutMin=[]  PCopyOutMax=[]  NCopyOutDataTypeStr=Inherit: Inherit via back propagation  NCopyOutMin=[]  NCopyOutMax=[]  IntegratorContinuousStateAttributes=''  IntegratorStateMustResolveToSignalObject=off  IntegratorRTWStateStorageClass=Auto  FilterContinuousStateAttributes=''  FilterStateMustResolveToSignalObject=off  FilterRTWStateStorageClass=Auto  ParallelPVariant=InternalParameters  IdealPVariant=Disabled  IVariant=InternalParameters  DVariant=Disabled  IntegratorVariant=Continuous  SatVariant=Disabled  AWVariant=Passthrough  PCopyVariant=Disabled  TRVariant=Disabled  FdbkBlocksVariant=Forward  IdealPFdbkVariant=Disabled  SatFdbkVariant=Disabled  DerivativeFilterVariant=Disabled  NVariant=Disabled  NCopyVariant=Disabled_SignalSpec  FilterICVariant=Disabled  IntegratorICVariant=InternalICs  ExternalResetVariant=Disabled  TRSumVariant=Passthrough  SumFdbkVariant=Disabled  SumVariant=Sum_PI  TsampFilterVariant=InternalTs  TsampNgainVariant=Passthrough  TsampIntegralVariant=Disabled_SignalSpec  ExternalSaturationOutDataTypeStr=Inherit: Same as second input  DerivativeSourceVariant=Disabled  PreIntVariant=InternalPreInt
  PID Controller4 : slpidlib/PID Controller  Controller=PI  Form=Parallel  TimeDomain=Continuous-time  UseExternalTs=off  SampleTime=-1  IntegratorMethod=Forward Euler  FilterMethod=Forward Euler  ControllerParametersSource=internal  P=40  I=80  UseKiTs=off  D=0  UseExternalDerivativeSource=off  N=100  UseFilter=on  TunerSelectOption=Transfer Function Based (PID Tuner App)  InitialConditionSource=internal  InitialConditionForIntegrator=0  InitialConditionForFilter=0  DifferentiatorICPrevScaledInput=0  ExternalReset=none  TrackingMode=off  Kt=1  LimitOutput=off  SatLimitsSource=internal  UpperSaturationLimit=120  LowerSaturationLimit=-120  LinearizeAsGain=on  AntiWindupMode=back-calculation  Kb=1  LimitIntegrator=off  UpperIntegratorSaturationLimit=inf  LowerIntegratorSaturationLimit=-inf  POutMin=[]  POutMax=[]  IOutMin=[]  IOutMax=[]  DOutMin=[]  DOutMax=[]  NOutMin=[]  NOutMax=[]  SumOutMin=[]  SumOutMax=[]  SaturationOutMin=[]  SaturationOutMax=[]  PParamMin=[]  PParamMax=[]  IParamMin=[]  IParamMax=[]  DParamMin=[]  DParamMax=[]  NParamMin=[]  NParamMax=[]  KbParamMin=[]  KbParamMax=[]  KtParamMin=[]  KtParamMax=[]  KbOutMin=[]  KbOutMax=[]  KtOutMin=[]  KtOutMax=[]  IntegratorOutMin=[]  IntegratorOutMax=[]  FilterOutMin=[]  FilterOutMax=[]  SumI1OutMin=[]  SumI1OutMax=[]  SumI2OutMin=[]  SumI2OutMax=[]  SumI3OutMin=[]  SumI3OutMax=[]  SumI4OutMin=[]  SumI4OutMax=[]  SumDOutMin=[]  SumDOutMax=[]  DifferentiatorOutMin=[]  DifferentiatorOutMax=[]  FilterDiffOutCoefMin=[]  FilterDiffOutCoefMax=[]  ReciprocalOutMin=[]  ReciprocalOutMax=[]  SumDenOutMin=[]  SumDenOutMax=[]  SumNumOutMin=[]  SumNumOutMax=[]  DivideOutMin=[]  DivideOutMax=[]  UdiffTsProdOutMin=[]  UdiffTsProdOutMax=[]  NTsProdOutMin=[]  NTsProdOutMax=[]  UintegralTsProdOutMin=[]  UintegralTsProdOutMax=[]  UngainTsProdOutMin=[]  UngainTsProdOutMax=[]  ClampingZeroOutDataTypeStr=Inherit: Inherit via back propagation  ClampingZeroOutMin=[]  ClampingZeroOutMax=[]  FilterDenConstantOutDataTypeStr=Inherit: Inherit via back propagation  FilterDenConstantOutMin=[]  FilterDenConstantOutMax=[]  PCopyOutDataTypeStr=Inherit: Inherit via back propagation  PCopyOutMin=[]  PCopyOutMax=[]  NCopyOutDataTypeStr=Inherit: Inherit via back propagation  NCopyOutMin=[]  NCopyOutMax=[]  IntegratorContinuousStateAttributes=''  IntegratorStateMustResolveToSignalObject=off  IntegratorRTWStateStorageClass=Auto  FilterContinuousStateAttributes=''  FilterStateMustResolveToSignalObject=off  FilterRTWStateStorageClass=Auto  ParallelPVariant=InternalParameters  IdealPVariant=Disabled  IVariant=InternalParameters  DVariant=Disabled  IntegratorVariant=Continuous  SatVariant=Disabled  AWVariant=Passthrough  PCopyVariant=Disabled  TRVariant=Disabled  FdbkBlocksVariant=Forward  IdealPFdbkVariant=Disabled  SatFdbkVariant=Disabled  DerivativeFilterVariant=Disabled  NVariant=Disabled  NCopyVariant=Disabled_SignalSpec  FilterICVariant=Disabled  IntegratorICVariant=InternalICs  ExternalResetVariant=Disabled  TRSumVariant=Passthrough  SumFdbkVariant=Disabled  SumVariant=Sum_PI  TsampFilterVariant=InternalTs  TsampNgainVariant=Passthrough  TsampIntegralVariant=Disabled_SignalSpec  ExternalSaturationOutDataTypeStr=Inherit: Same as second input  DerivativeSourceVariant=Disabled  PreIntVariant=InternalPreInt
  PID Controller6 : slpidlib/PID Controller  Controller=PI  Form=Parallel  TimeDomain=Continuous-time  UseExternalTs=off  SampleTime=-1  IntegratorMethod=Forward Euler  FilterMethod=Forward Euler  ControllerParametersSource=internal  P=-15  I=-75  UseKiTs=off  D=0  UseExternalDerivativeSource=off  N=100  UseFilter=on  TunerSelectOption=Transfer Function Based (PID Tuner App)  InitialConditionSource=internal  InitialConditionForIntegrator=0  InitialConditionForFilter=0  DifferentiatorICPrevScaledInput=0  ExternalReset=none  TrackingMode=off  Kt=1  LimitOutput=off  SatLimitsSource=internal  UpperSaturationLimit=500  LowerSaturationLimit=-500  LinearizeAsGain=on  AntiWindupMode=back-calculation  Kb=1  LimitIntegrator=off  UpperIntegratorSaturationLimit=inf  LowerIntegratorSaturationLimit=-inf  POutMin=[]  POutMax=[]  IOutMin=[]  IOutMax=[]  DOutMin=[]  DOutMax=[]  NOutMin=[]  NOutMax=[]  SumOutMin=[]  SumOutMax=[]  SaturationOutMin=[]  SaturationOutMax=[]  PParamMin=[]  PParamMax=[]  IParamMin=[]  IParamMax=[]  DParamMin=[]  DParamMax=[]  NParamMin=[]  NParamMax=[]  KbParamMin=[]  KbParamMax=[]  KtParamMin=[]  KtParamMax=[]  KbOutMin=[]  KbOutMax=[]  KtOutMin=[]  KtOutMax=[]  IntegratorOutMin=[]  IntegratorOutMax=[]  FilterOutMin=[]  FilterOutMax=[]  SumI1OutMin=[]  SumI1OutMax=[]  SumI2OutMin=[]  SumI2OutMax=[]  SumI3OutMin=[]  SumI3OutMax=[]  SumI4OutMin=[]  SumI4OutMax=[]  SumDOutMin=[]  SumDOutMax=[]  DifferentiatorOutMin=[]  DifferentiatorOutMax=[]  FilterDiffOutCoefMin=[]  FilterDiffOutCoefMax=[]  ReciprocalOutMin=[]  ReciprocalOutMax=[]  SumDenOutMin=[]  SumDenOutMax=[]  SumNumOutMin=[]  SumNumOutMax=[]  DivideOutMin=[]  DivideOutMax=[]  UdiffTsProdOutMin=[]  UdiffTsProdOutMax=[]  NTsProdOutMin=[]  NTsProdOutMax=[]  UintegralTsProdOutMin=[]  UintegralTsProdOutMax=[]  UngainTsProdOutMin=[]  UngainTsProdOutMax=[]  ClampingZeroOutDataTypeStr=Inherit: Inherit via back propagation  ClampingZeroOutMin=[]  ClampingZeroOutMax=[]  FilterDenConstantOutDataTypeStr=Inherit: Inherit via back propagation  FilterDenConstantOutMin=[]  FilterDenConstantOutMax=[]  PCopyOutDataTypeStr=Inherit: Inherit via back propagation  PCopyOutMin=[]  PCopyOutMax=[]  NCopyOutDataTypeStr=Inherit: Inherit via back propagation  NCopyOutMin=[]  NCopyOutMax=[]  IntegratorContinuousStateAttributes=''  IntegratorStateMustResolveToSignalObject=off  IntegratorRTWStateStorageClass=Auto  FilterContinuousStateAttributes=''  FilterStateMustResolveToSignalObject=off  FilterRTWStateStorageClass=Auto  ParallelPVariant=InternalParameters  IdealPVariant=Disabled  IVariant=InternalParameters  DVariant=Disabled  IntegratorVariant=Continuous  SatVariant=Disabled  AWVariant=Passthrough  PCopyVariant=Disabled  TRVariant=Disabled  FdbkBlocksVariant=Forward  IdealPFdbkVariant=Disabled  SatFdbkVariant=Disabled  DerivativeFilterVariant=Disabled  NVariant=Disabled  NCopyVariant=Disabled_SignalSpec  FilterICVariant=Disabled  IntegratorICVariant=InternalICs  ExternalResetVariant=Disabled  TRSumVariant=Passthrough  SumFdbkVariant=Disabled  SumVariant=Sum_PI  TsampFilterVariant=InternalTs  TsampNgainVariant=Passthrough  TsampIntegralVariant=Disabled_SignalSpec  ExternalSaturationOutDataTypeStr=Inherit: Same as second input  DerivativeSourceVariant=Disabled  PreIntVariant=InternalPreInt
  ParkClarke : MATLAB Function  TreatAsAtomicUnit=on
  Product : Product
  Selector : Selector  InputPortWidth=5  IndexOptions=Index vector (dialog)  Indices=[5]  OutputSizes=1
  Selector1 : Selector  InputPortWidth=5  IndexOptions=Index vector (dialog)  Indices=[4]  OutputSizes=1
  Selector2 : Selector  InputPortWidth=5  IndexOptions=Index vector (dialog)  Indices=[1:3]  OutputSizes=1
  To File : ToFile  Commented=on  Filename=SimData\SteeringVabc.mat  SaveFormat=Timeseries
  Unit Delay : UnitDelay  InitialCondition=[0;0]  SampleTime=-1  HasFrameUpgradeWarning=on
  Vabc : Scope  NumInputPorts=3
  Wm_abc : Scope
  theta_abc : Scope
  dd_ctrl : Outport
  wires:
  Constant4/1 -> Add3/1  "i_d_ref"
  Back EMF/1(Fabc) -> BLDC abc model/2(f)
  Unit Delay/1 -> Demux1/1
  Add11/1 -> PID Controller6/1, [err_PI2]
  Add9/1 -> [err_PI1], PID Controller10/1
  Demux1/2 -> [I_q], Add4/2
  [Wm_abc] -> Add11/2
  [Theta_abc] -> Add9/2
  Selector2/1 -> ParkClarke/1(X_abc), I_abc/1, [I_abc]  "I_abc"
  Mux1/1 -> InvParkClarke/1(X_dq)
  [Theta_abc] -> ParkClarke/2(theta)
  [Theta_abc] -> InvParkClarke/2(theta)
  Selector/1 -> [Theta_abc], Divide/1  "Theta_abc"
  PID Controller3/1 -> Mux1/1
  ParkClarke/1(Y_dq) -> Unit Delay/1
  Constant1/1 -> BLDC abc model/4(Tl)
  InvParkClarke/1(Y_abc) -> BLDC abc model/3(v), To File/1, Demux2/1  "Vabc"
  PID Controller4/1 -> Mux1/2
  BLDC abc model/1(dX) -> Integrator2/1
  Selector1/1 -> [Wm_abc], Wm_abc/1  "Wm_abc"
  Add4/1 -> [err_PI3], PID Controller4/1
  Demux1/1 -> [I_d], Add3/2
  Add3/1 -> PID Controller3/1, [err_PI4]
  Integrator2/1 -> Selector2/1, Selector/1, Selector1/1, BLDC abc model/1(X), Back EMF/1(X)
  [i_q_ref] -> Add4/1
  Product/1 -> Add9/1
  dd_ref/1 -> Product/1  "dd_ref"
  Constant2/1 -> Product/2
  Divide/1 -> dd_ctrl/1
  Constant3/1 -> Divide/2
  [I_d] -> Idq/1
  [I_q] -> Idq/2
  [err_PI1] -> PI errors/1
  [err_PI2] -> PI errors/2
  [err_PI3] -> PI errors/3
  [err_PI4] -> PI errors/4
  Demux2/1 -> Vabc/1
  Demux2/2 -> Vabc/2
  Demux2/3 -> Vabc/3
  PID Controller6/1 -> [i_q_ref]  "i_q_ref"
  PID Controller10/1 -> Add11/1  "i_d_ref"

== system LongLatDriveline/SteerActuator/NoActuator ==
  dd_ref : Inport
  dd_ctrl : Outport
  wires:
  dd_ref/1 -> dd_ctrl/1

== system LongLatDriveline/SteerActuator/genericTransferFunction ==
  dd_ref : Inport
  TF_AlcalaUrbano : TransferFcn  Commented=on  Numerator=[(2*pi*5)^2]  Denominator=[1 2*0.7*(2*pi*5) (2*pi*5)^2]
  TF_BLDCIdentification : TransferFcn  Numerator=1552  Denominator=[1 18.95 1543]
  dd_ctrl : Outport
  wires:
  dd_ref/1 -> TF_BLDCIdentification/1
  TF_BLDCIdentification/1 -> dd_ctrl/1
